simulink library "DAEMOT_Lib"  (R2019b)
settings: Solver=ode45  StartTime=0.0  StopTime=10.0  FixedStep=0.1  RelTol=1e-3
undefined symbols (not defined in the file or in its folder): Controller, CP, Ctrl, Ctrl_Fcn, Elec1, f, F2, Fluid, lag1, Mission, Moody, PropellerProp, rev_comms_sink
libraries: $bdroot x200, instrumentlib x21, simulink x5, dspsigops x2
(part 7 of 13)

== system DAEMOT_Lib/Electrical/Air Vehicle ==
  In1 : Inport
  Bus Creator2 : BusCreator  Inputs=4
  Bus Selector2 : BusSelector  OutputSignals=aspeed,torque
  Constant : Constant  Value=theta
  Data_Sink : Subsystem  LoadFcn=|  InitFcn=|  mask(Data Sink){}
      LoadFcn=|
      | h      = get_param(gcb,'handle');   % Get block handle                           
      | hblock = get(h);     % Parse out handles structure
      | 
      | str = [hblock.Path(numel(bdroot)+2:end), hblock.Name];
      | str(~ismember(str,['A':'Z' 'a':'z' '0':'9' '_'])) = '';                     
      | set_param([gcb, '/global_data_goto'],'GotoTag',['gdata_',str]);
      |                                
      |                                                                                  
      | clear h hblock str
      InitFcn=|
      | h      = get_param(gcb,'handle');   % Get block handle                           
      | hblock = get(h);     % Parse out handles structure
      | 
      | str = [hblock.Path(numel(bdroot)+2:end), hblock.Name];
      | str(~ismember(str,['A':'Z' 'a':'z' '0':'9' '_'])) = '';                     
      | set_param([gcb, '/global_data_goto'],'GotoTag',['gdata_',str]);
      |                                
      |                                                                                  
      | clear h hblock str
      mask help:
      | Input to this block should be a bus signal with named signals.
      |
      | Bus signals sent to this block will be read by the Data Manager.
      | The Data Manager will handle the global routing of signals.
      |
      | This block should be placed under the mask of components.
      settings: CopyFcn=|
      | h      = get_param(gcb,'handle');   % Get block handle
      | hblock = get(h);     % Parse out handles structure
      | 
      | str = [hblock.Path(numel(bdroot)+2:end), hblock.Name];
      | str(~ismember(str,['A':'Z' 'a':'z' '0':'9' '_'])) = '';
      | set_param([gcb, '/global_data_goto'],'GotoTag',['gdata_',str]);
      | 
      | 
      | clear h hblock str
      settings: NameChangeFcn=|
      | h      = get_param(gcb,'handle');   % Get block handle
      | hblock = get(h);     % Parse out handles structure
      | 
      | str = [hblock.Path(numel(bdroot)+2:end), hblock.Name];
      | str(~ismember(str,['A':'Z' 'a':'z' '0':'9' '_'])) = '';
      | set_param([gcb, '/global_data_goto'],'GotoTag',['gdata_',str]);
      | 
      | 
      | clear h hblock str
      mask Display: text(0.25,0.5,'Data Sink')
  Fcn : Fcn  Expr=u(1)*cos(u(2))
  Fcn1 : Fcn  Expr=u(1)*sin(u(2))
  Integrator : Integrator  InitialCondition=v_initial
  Mux : Mux  Inputs=2
  Sink1 : Subsystem  LoadFcn=rev_comms_sink();  InitFcn=rev_comms_sink();  mask(Sink){}
      mask help: Used for sending data to the upstream component.
      settings: CopyFcn=rev_comms_sink();  NameChangeFcn=rev_comms_sink();
      mask Display: text(0.25,0.5,'Sink')
  Terminator1 : Terminator
  speed : MATLAB Function  TreatAsAtomicUnit=on
  wires:
  Constant/1 -> Mux/2
  [v] -> Mux/1
  Mux/1 -> Fcn/1, Fcn1/1
  Fcn1/1 -> Bus Creator2/4  "Vertical Speed [m_s]"
  Fcn/1 -> Bus Creator2/3  "Lateral Speed [m_s]"
  speed/2(tau) -> [tau]
  speed/1(v_dot) -> Integrator/1
  [omega] -> speed/2(omega)
  [tau] -> Bus Creator2/1  "Load Torque [Nm]"
  Bus Creator2/1 -> Data_Sink/1(" ")
  [v] -> Bus Creator2/2  "Vehicle Speed [m_s]"
  Bus Selector2/2 -> Terminator1/1  "<torque>"
  In1/1 -> Bus Selector2/1
  Bus Selector2/1 -> [omega]  "<aspeed>"
  [tau] -> Sink1/1(In1)
  Integrator/1 -> [v]
  [v] -> speed/1(v)

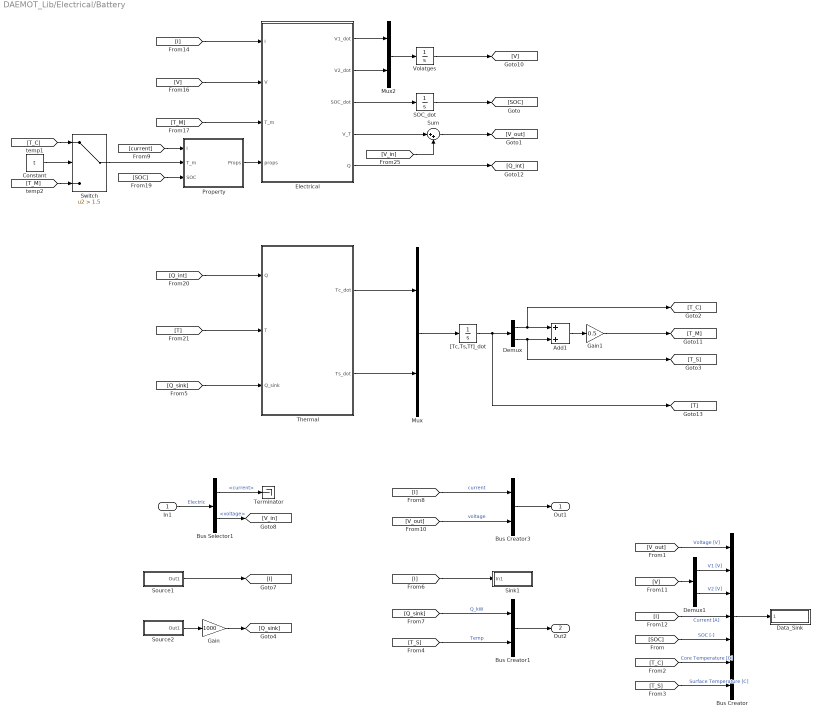
== system DAEMOT_Lib/Electrical/Battery ==
  In1 : Inport
  Add1 : Sum
  Bus Creator : BusCreator  Inputs=7
  Bus Creator1 : BusCreator  Inputs=2
  Bus Creator3 : BusCreator  Inputs=2
  Bus Selector1 : BusSelector  OutputSignals=current,voltage
  Constant : Constant  Value=t
  Data_Sink : Subsystem  LoadFcn=|  InitFcn=|  mask(Data Sink){}
      LoadFcn=|
      | h      = get_param(gcb,'handle');   % Get block handle                           
      | hblock = get(h);     % Parse out handles structure
      | 
      | str = [hblock.Path(numel(bdroot)+2:end), hblock.Name];
      | str(~ismember(str,['A':'Z' 'a':'z' '0':'9' '_'])) = '';                     
      | set_param([gcb, '/global_data_goto'],'GotoTag',['gdata_',str]);
      |                                
      |                                                                                  
      | clear h hblock str
      InitFcn=|
      | h      = get_param(gcb,'handle');   % Get block handle                           
      | hblock = get(h);     % Parse out handles structure
      | 
      | str = [hblock.Path(numel(bdroot)+2:end), hblock.Name];
      | str(~ismember(str,['A':'Z' 'a':'z' '0':'9' '_'])) = '';                     
      | set_param([gcb, '/global_data_goto'],'GotoTag',['gdata_',str]);
      |                                
      |                                                                                  
      | clear h hblock str
      mask help:
      | Input to this block should be a bus signal with named signals.
      |
      | Bus signals sent to this block will be read by the Data Manager.
      | The Data Manager will handle the global routing of signals.
      |
      | This block should be placed under the mask of components.
      settings: CopyFcn=|
      | h      = get_param(gcb,'handle');   % Get block handle
      | hblock = get(h);     % Parse out handles structure
      | 
      | str = [hblock.Path(numel(bdroot)+2:end), hblock.Name];
      | str(~ismember(str,['A':'Z' 'a':'z' '0':'9' '_'])) = '';
      | set_param([gcb, '/global_data_goto'],'GotoTag',['gdata_',str]);
      | 
      | 
      | clear h hblock str
      settings: NameChangeFcn=|
      | h      = get_param(gcb,'handle');   % Get block handle
      | hblock = get(h);     % Parse out handles structure
      | 
      | str = [hblock.Path(numel(bdroot)+2:end), hblock.Name];
      | str(~ismember(str,['A':'Z' 'a':'z' '0':'9' '_'])) = '';
      | set_param([gcb, '/global_data_goto'],'GotoTag',['gdata_',str]);
      | 
      | 
      | clear h hblock str
      mask Display: text(0.25,0.5,'Data Sink')
  Demux : Demux  Outputs=2
  Demux1 : Demux  Outputs=2
  Electrical : MATLAB Function  TreatAsAtomicUnit=on
  Gain : Gain  Gain=1000
  Gain1 : Gain  Gain=0.5
  Mux : Mux  Inputs=2
  Mux2 : Mux  Inputs=2
  Property : Subsystem
  SOC_dot : Integrator  InitialCondition=SOC_initial
  Sink1 : Subsystem  LoadFcn=rev_comms_sink();  InitFcn=rev_comms_sink();  mask(Sink){}
      mask help: Used for sending data to the upstream component.
      settings: CopyFcn=rev_comms_sink();  NameChangeFcn=rev_comms_sink();
      mask Display: text(0.25,0.5,'Sink')
  Source1 : Subsystem  mask(Source){}
      mask help: Used for receiving data from the downstream component.
      mask init:
      | n_src = gcb;
      | n_src = str2num(n_src(end));
      | try
      |     rev_comms_source(n_src);
      | catch
      | 
      | end
      mask Display: text(0.25,0.5,'Source')
  Source2 : Subsystem  mask(Source){}
      mask help: Used for receiving data from the downstream component.
      mask init:
      | n_src = gcb;
      | n_src = str2num(n_src(end));
      | try
      |     rev_comms_source(n_src);
      | catch
      | 
      | end
      mask Display: text(0.25,0.5,'Source')
  Sum : Sum  Inputs=|++
  Switch : Switch  Criteria=u2 > Threshold  Threshold=1.5
  Terminator : Terminator
  Thermal : MATLAB Function  TreatAsAtomicUnit=on
  Volatges : Integrator  InitialCondition=RC_initial
  "[Tc,Ts,Tf]_dot" : Integrator  InitialCondition=[Tc_initial, Ts_initial]
  Out1 : Outport
  Out2 : Outport  Port=2
  wires:
  [I] -> Bus Creator/4  "Current [A]"
  [V] -> Demux1/1
  Demux1/1 -> Bus Creator/2  "V1 [V]"
  Demux1/2 -> Bus Creator/3  "V2 [V]"
  Switch/1 -> Property/2(T_m)
  [T_M] -> Switch/3
  [T_C] -> Switch/1
  Constant/1 -> Switch/2
  Electrical/2(V2_dot) -> Mux2/2
  Electrical/1(V1_dot) -> Mux2/1
  Electrical/3(SOC_dot) -> SOC_dot/1
  Sum/1 -> [V_out]
  Electrical/4(V_T) -> Sum/1
  [V_in] -> Sum/2
  Electrical/5(Q) -> [Q_int]
  Property/1(Props) -> Electrical/4(props)
  [V] -> Electrical/2(V)
  [T_M] -> Electrical/3(T_m)
  [I] -> Electrical/1(I)
  Mux2/1 -> Volatges/1
  Demux/2 -> [T_S], Add1/2
  Demux/1 -> [T_C], Add1/1
  "[Tc,Ts,Tf]_dot"/1 -> [T], Demux/1
  SOC_dot/1 -> [SOC]
  Volatges/1 -> [V]
  Add1/1 -> Gain1/1
  Mux/1 -> "[Tc,Ts,Tf]_dot"/1
  [SOC] -> Bus Creator/5  "SOC [-]"
  [V_out] -> Bus Creator/1  "Voltage [V]"
  [T_C] -> Bus Creator/6  "Core Temperature [C]"
  [T_S] -> Bus Creator/7  "Surface Temperature [C]"
  In1/1 -> Bus Selector1/1  "Electric"
  Bus Creator3/1 -> Out1/1
  [I] -> Bus Creator3/1  "current"
  Bus Selector1/1 -> Terminator/1  "<current>"
  Bus Selector1/2 -> [V_in]  "<voltage>"
  [V_out] -> Bus Creator3/2  "voltage"
  [current] -> Property/1(I)
  Gain1/1 -> [T_M]
  Bus Creator/1 -> Data_Sink/1(" ")
  [SOC] -> Property/3(SOC)
  [Q_int] -> Thermal/1(Q)
  [T] -> Thermal/2(T)
  Thermal/1(Tc_dot) -> Mux/1
  Thermal/2(Ts_dot) -> Mux/2
  [Q_sink] -> Thermal/3(Q_sink)
  Source2/1(Out1) -> Gain/1
  [I] -> Sink1/1(In1)
  Source1/1(Out1) -> [I]
  Bus Creator1/1 -> Out2/1
  [T_S] -> Bus Creator1/2  "Temp"
  [Q_sink] -> Bus Creator1/1  "Q_kW"
  Gain/1 -> [Q_sink]

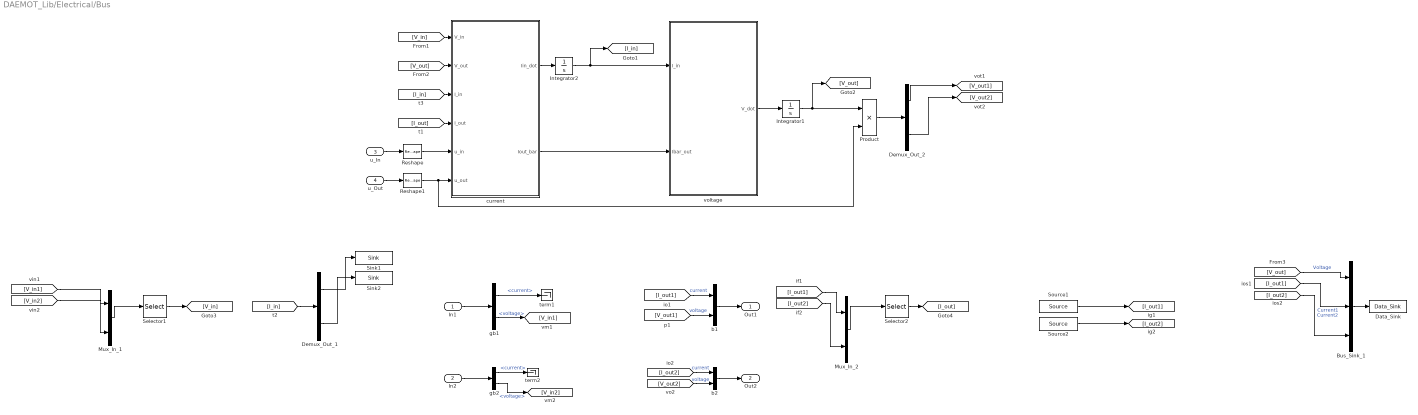
== system DAEMOT_Lib/Electrical/Bus ==
  In1 : Inport
  In2 : Inport  Port=2
  u_In : Inport  Port=3
  u_Out : Inport  Port=4
  Bus_Sink_1 : BusCreator  Inputs=3
  Data_Sink : $bdroot/Support Functions/Data_Sink
  Demux_Out_1 : Demux  Outputs=2
  Demux_Out_2 : Demux  Outputs=2
  Integrator1 : Integrator  InitialCondition=V_initial
  Integrator2 : Integrator  InitialCondition=I_initial*ones(Num_In,1)
  Mux_In_1 : Mux  Inputs=2
  Mux_In_2 : Mux  Inputs=2
  Product : Product
  Reshape : Reshape
  Reshape1 : Reshape
  Selector1 : Selector  InputPortWidth=2  IndexOptions=Index vector (dialog)  Indices=[1 2 ]  OutputSizes=1
  Selector2 : Selector  InputPortWidth=2  IndexOptions=Index vector (dialog)  Indices=[1 2 ]  OutputSizes=1
  Sink1 : $bdroot/Support Functions/Sink
  Sink2 : $bdroot/Support Functions/Sink
  Source1 : $bdroot/Support Functions/Source
  Source2 : $bdroot/Support Functions/Source
  b1 : BusCreator  Inputs=2
  b2 : BusCreator  Inputs=2
  current : MATLAB Function  TreatAsAtomicUnit=on
  gb1 : BusSelector  OutputSignals=current,voltage
  gb2 : BusSelector  OutputSignals=current,voltage
  term1 : Terminator
  term2 : Terminator
  voltage : MATLAB Function  TreatAsAtomicUnit=on
  Out1 : Outport  VectorParamsAs1DForOutWhenUnconnected=off
  Out2 : Outport  Port=2  VectorParamsAs1DForOutWhenUnconnected=off
  wires:
  Demux_Out_1/1 -> Sink1/1
  [V_in1] -> Mux_In_1/1
  gb1/2 -> [V_in1]  "<voltage>"
  gb1/1 -> term1/1  "<current>"
  In1/1 -> gb1/1
  [I_in] -> Demux_Out_1/1
  Integrator2/1 -> voltage/1(I_in), [I_in]
  voltage/1(V_dot) -> Integrator1/1
  Integrator1/1 -> Product/1, [V_out]
  [V_out] -> current/2(V_out)
  Mux_In_1/1 -> Selector1/1
  current/1(Iin_dot) -> Integrator2/1
  [I_in] -> current/3(I_in)
  u_In/1 -> Reshape/1
  Demux_Out_2/1 -> [V_out1]
  Bus_Sink_1/1 -> Data_Sink/1
  [I_out1] -> Mux_In_2/1
  Mux_In_2/1 -> Selector2/1
  [V_out1] -> b1/2  "voltage"
  [I_out1] -> b1/1  "current"
  Source1/1 -> [I_out1]
  b1/1 -> Out1/1
  u_Out/1 -> Reshape1/1
  current/2(Iout_bar) -> voltage/2(Ibar_out)
  Product/1 -> Demux_Out_2/1
  [V_in] -> current/1(V_in)
  Selector1/1 -> [V_in]
  In2/1 -> gb2/1
  gb2/2 -> [V_in2]  "<voltage>"
  gb2/1 -> term2/1  "<current>"
  Demux_Out_1/2 -> Sink2/1
  [V_in2] -> Mux_In_1/2
  [I_out] -> current/4(I_out)
  Selector2/1 -> [I_out]
  [V_out] -> Bus_Sink_1/1  "Voltage"
  [I_out1] -> Bus_Sink_1/2  "Current1"
  [I_out2] -> b2/1  "current"
  [V_out2] -> b2/2  "voltage"
  [I_out2] -> Bus_Sink_1/3  "Current2"
  b2/1 -> Out2/1
  Source2/1 -> [I_out2]
  [I_out2] -> Mux_In_2/2
  Demux_Out_2/2 -> [V_out2]
  Reshape/1 -> current/5(u_in)
  Reshape1/1 -> Product/2, current/6(u_out)

== system DAEMOT_Lib/Electrical/Capacitor ==
  In1 : Inport
  Bus Creator1 : BusCreator  Inputs=1
  Bus Creator3 : BusCreator  Inputs=2
  Bus Selector1 : BusSelector  OutputSignals=current,voltage
  Data_Sink : $bdroot/Support Functions/Data_Sink
  Integrator2 : Integrator  InitialCondition=V_initial
  Sink1 : $bdroot/Support Functions/Sink
  Source1 : $bdroot/Support Functions/Source
  Terminator : Terminator
  Voltage : MATLAB Function  TreatAsAtomicUnit=on
  Out1 : Outport  VectorParamsAs1DForOutWhenUnconnected=off
  wires:
  Integrator2/1 -> [V]
  [Current_out] -> Bus Creator3/1  "current"
  Bus Selector1/1 -> [Current_in]  "<current>"
  Bus Selector1/2 -> Terminator/1  "<voltage>"
  [V] -> Bus Creator3/2  "voltage"
  [V] -> Sink1/1
  In1/1 -> Bus Selector1/1  "electric"
  [Current_out] -> Voltage/2(I_out)
  Bus Creator3/1 -> Out1/1
  Voltage/1(V_dot) -> Integrator2/1
  [Current_in] -> Voltage/1(I_in)
  [V] -> Bus Creator1/1  "Voltage"
  Bus Creator1/1 -> Data_Sink/1
  Source1/1 -> [Current_out]

== system DAEMOT_Lib/Electrical/Converter ==
  In1 : Inport
  In2 : Inport  Port=2
  In3 : Inport  Port=3
  Bus Creator1 : BusCreator  Inputs=2
  Bus Creator2 : BusCreator  Inputs=3
  Bus Creator3 : BusCreator  Inputs=2
  Bus Selector1 : BusSelector  OutputSignals=current,voltage
  Current : MATLAB Function  TreatAsAtomicUnit=on
  Data_Sink : $bdroot/Support Functions/Data_Sink
  Gain : Gain  Gain=1000
  Integrator1 : Integrator  InitialCondition=T_initial
  Scope : Scope
  Sink1 : $bdroot/Support Functions/Sink
  Source1 : $bdroot/Support Functions/Source
  Source2 : $bdroot/Support Functions/Source
  Terminator : Terminator
  Thermal : MATLAB Function  TreatAsAtomicUnit=on
  Voltage : MATLAB Function  TreatAsAtomicUnit=on
  Out1 : Outport  VectorParamsAs1DForOutWhenUnconnected=off
  Out2 : Outport  Port=2  VectorParamsAs1DForOutWhenUnconnected=off
  wires:
  Source2/1 -> Gain/1
  Voltage/2(Q) -> Scope/1, [Q]
  [I_out] -> Voltage/3(I_out)
  [T] -> Bus Creator2/3  "Temperature"
  [I_out] -> Bus Creator2/1  "Current"
  [V_out] -> Bus Creator2/2  "Voltage"
  Bus Creator2/1 -> Data_Sink/1
  Thermal/1(T_dot) -> Integrator1/1
  Integrator1/1 -> [T]
  [Q] -> Thermal/1(Q)
  [Q_sink] -> Thermal/2(Q_sink)
  In3/1 -> Current/3(s), Voltage/5(s)
  In2/1 -> Current/2(D), Voltage/4(D)
  Current/1(I_in) -> [I_in], Voltage/2(I_in)
  [I_out] -> Current/1(I_out)
  Voltage/1(V_out) -> [V_out]
  [V_in] -> Voltage/1(V_in)
  [I_out] -> Bus Creator3/1  "current"
  Source1/1 -> [I_out]
  Bus Selector1/1 -> Terminator/1  "<current>"
  Bus Selector1/2 -> [V_in]  "<voltage>"
  [V_out] -> Bus Creator3/2  "voltage"
  In1/1 -> Bus Selector1/1  "electric"
  Bus Creator3/1 -> Out1/1
  [I_in] -> Sink1/1
  Bus Creator1/1 -> Out2/1
  [T] -> Bus Creator1/2  "Temp"
  [Q_sink] -> Bus Creator1/1  "Q_kW"
  Gain/1 -> [Q_sink]

== system DAEMOT_Lib/Electrical/Cooling Sink ==
  In1 : Inport
  In2 : Inport  Port=2
  Sink1 : $bdroot/Support Functions/Sink
  Terminator : Terminator
  wires:
  In1/1 -> Terminator/1
  In2/1 -> Sink1/1  "Q_kW"

== system DAEMOT_Lib/Electrical/Cooling Source ==
  In1 : Inport
  Constant : Constant
  Source1 : $bdroot/Support Functions/Source
  Terminator : Terminator
  b1 : BusCreator  Inputs=2
  Out1 : Outport  VectorParamsAs1DForOutWhenUnconnected=off
  wires:
  In1/1 -> b1/1  "Q_kW"
  b1/1 -> Out1/1
  Constant/1 -> b1/2  "Temp"
  Source1/1 -> Terminator/1

== system DAEMOT_Lib/Electrical/Current Sink ==
  In1 : Inport
  In2 : Inport  Port=2
  Sink1 : Subsystem  LoadFcn=rev_comms_sink();  InitFcn=rev_comms_sink();  mask(Sink){}
      mask help: Used for sending data to the upstream component.
      settings: CopyFcn=rev_comms_sink();  NameChangeFcn=rev_comms_sink();
      mask Display: text(0.25,0.5,'Sink')
  Terminator : Terminator
  wires:
  In1/1 -> Terminator/1
  In2/1 -> Sink1/1(In1)  "current"

== system DAEMOT_Lib/Electrical/Current Source ==
  In1 : Inport
  Constant : Constant  Value=0
  Source1 : Subsystem  mask(Source){}
      mask help: Used for receiving data from the downstream component.
      mask init:
      | n_src = gcb;
      | n_src = str2num(n_src(end));
      | try
      |     rev_comms_source(n_src);
      | catch
      | 
      | end
      mask Display: text(0.25,0.5,'Source')
  Terminator : Terminator
  b1 : BusCreator  Inputs=2
  Out1 : Outport  VectorParamsAs1DForOutWhenUnconnected=off
  wires:
  b1/1 -> Out1/1
  Constant/1 -> b1/2  "voltage"
  Source1/1(Out1) -> Terminator/1
  In1/1 -> b1/1  "current"

== system DAEMOT_Lib/Electrical/ESC ==
  In1 : Inport
  Bus Creator2 : BusCreator  Inputs=1
  Bus Selector2 : BusSelector  OutputSignals=current,voltage
  Data_Sink : Subsystem  LoadFcn=|  InitFcn=|  mask(Data Sink){}
      LoadFcn=|
      | h      = get_param(gcb,'handle');   % Get block handle                           
      | hblock = get(h);     % Parse out handles structure
      | 
      | str = [hblock.Path(numel(bdroot)+2:end), hblock.Name];
      | str(~ismember(str,['A':'Z' 'a':'z' '0':'9' '_'])) = '';                     
      | set_param([gcb, '/global_data_goto'],'GotoTag',['gdata_',str]);
      |                                
      |                                                                                  
      | clear h hblock str
      InitFcn=|
      | h      = get_param(gcb,'handle');   % Get block handle                           
      | hblock = get(h);     % Parse out handles structure
      | 
      | str = [hblock.Path(numel(bdroot)+2:end), hblock.Name];
      | str(~ismember(str,['A':'Z' 'a':'z' '0':'9' '_'])) = '';                     
      | set_param([gcb, '/global_data_goto'],'GotoTag',['gdata_',str]);
      |                                
      |                                                                                  
      | clear h hblock str
      mask help:
      | Input to this block should be a bus signal with named signals.
      |
      | Bus signals sent to this block will be read by the Data Manager.
      | The Data Manager will handle the global routing of signals.
      |
      | This block should be placed under the mask of components.
      settings: CopyFcn=|
      | h      = get_param(gcb,'handle');   % Get block handle
      | hblock = get(h);     % Parse out handles structure
      | 
      | str = [hblock.Path(numel(bdroot)+2:end), hblock.Name];
      | str(~ismember(str,['A':'Z' 'a':'z' '0':'9' '_'])) = '';
      | set_param([gcb, '/global_data_goto'],'GotoTag',['gdata_',str]);
      | 
      | 
      | clear h hblock str
      settings: NameChangeFcn=|
      | h      = get_param(gcb,'handle');   % Get block handle
      | hblock = get(h);     % Parse out handles structure
      | 
      | str = [hblock.Path(numel(bdroot)+2:end), hblock.Name];
      | str(~ismember(str,['A':'Z' 'a':'z' '0':'9' '_'])) = '';
      | set_param([gcb, '/global_data_goto'],'GotoTag',['gdata_',str]);
      | 
      | 
      | clear h hblock str
      mask Display: text(0.25,0.5,'Data Sink')
  Polynomial : Polyval  Coefs=Esc.coeffs
  Sink1 : Subsystem  LoadFcn=rev_comms_sink();  InitFcn=rev_comms_sink();  mask(Sink){}
      mask help: Used for sending data to the upstream component.
      settings: CopyFcn=rev_comms_sink();  NameChangeFcn=rev_comms_sink();
      mask Display: text(0.25,0.5,'Sink')
  Terminator1 : Terminator
  wires:
  [current] -> Sink1/1(In1)
  Bus Selector2/2 -> [voltage]  "<voltage>"
  In1/1 -> Bus Selector2/1
  Bus Creator2/1 -> Data_Sink/1(" ")
  [current] -> Bus Creator2/1  "Current Load [A]"
  Bus Selector2/1 -> Terminator1/1  "<current>"
  [voltage] -> Polynomial/1
  Polynomial/1 -> [current]

== system DAEMOT_Lib/Electrical/Effort Sink ==
  In1 : Inport
  Sink1 : Subsystem  LoadFcn=rev_comms_sink();  InitFcn=rev_comms_sink();  mask(Sink){}
      mask help: Used for sending data to the upstream component.
      settings: CopyFcn=rev_comms_sink();  NameChangeFcn=rev_comms_sink();
      mask Display: text(0.25,0.5,'Sink')
  Terminator : Terminator
  val : Constant  Value=value
  wires:
  val/1 -> Sink1/1(In1)
  In1/1 -> Terminator/1

== system DAEMOT_Lib/Electrical/Effort Source ==
  Constant : Constant  Value=0
  Source1 : Subsystem  mask(Source){}
      mask help: Used for receiving data from the downstream component.
      mask init:
      | n_src = gcb;
      | n_src = str2num(n_src(end));
      | try
      |     rev_comms_source(n_src);
      | catch
      | 
      | end
      mask Display: text(0.25,0.5,'Source')
  Terminator : Terminator
  b1 : BusCreator  Inputs=2
  val : Constant  Value=value
  Out1 : Outport  VectorParamsAs1DForOutWhenUnconnected=off
  wires:
  val/1 -> b1/2  "voltage"
  Constant/1 -> b1/1  "current"
  Source1/1(Out1) -> Terminator/1
  b1/1 -> Out1/1

== system DAEMOT_Lib/Electrical/Engine ==
  In1 : Inport
  In2 : Inport  Port=2
  Bus Creator1 : BusCreator  Inputs=2
  Bus Selector1 : BusSelector  OutputSignals=current,voltage
  Compare To Constant : simulink/Logic and Bit Operations/Compare To Constant  relop=>  const=.01  OutDataTypeStr=uint8
  Constant : Constant  Value=0
  Data_Sink : Subsystem  LoadFcn=|  InitFcn=|  mask(Data Sink){}
      LoadFcn=|
      | h      = get_param(gcb,'handle');   % Get block handle                           
      | hblock = get(h);     % Parse out handles structure
      | 
      | str = [hblock.Path(numel(bdroot)+2:end), hblock.Name];
      | str(~ismember(str,['A':'Z' 'a':'z' '0':'9' '_'])) = '';                     
      | set_param([gcb, '/global_data_goto'],'GotoTag',['gdata_',str]);
      |                                
      |                                                                                  
      | clear h hblock str
      InitFcn=|
      | h      = get_param(gcb,'handle');   % Get block handle                           
      | hblock = get(h);     % Parse out handles structure
      | 
      | str = [hblock.Path(numel(bdroot)+2:end), hblock.Name];
      | str(~ismember(str,['A':'Z' 'a':'z' '0':'9' '_'])) = '';                     
      | set_param([gcb, '/global_data_goto'],'GotoTag',['gdata_',str]);
      |                                
      |                                                                                  
      | clear h hblock str
      mask help:
      | Input to this block should be a bus signal with named signals.
      |
      | Bus signals sent to this block will be read by the Data Manager.
      | The Data Manager will handle the global routing of signals.
      |
      | This block should be placed under the mask of components.
      settings: CopyFcn=|
      | h      = get_param(gcb,'handle');   % Get block handle
      | hblock = get(h);     % Parse out handles structure
      | 
      | str = [hblock.Path(numel(bdroot)+2:end), hblock.Name];
      | str(~ismember(str,['A':'Z' 'a':'z' '0':'9' '_'])) = '';
      | set_param([gcb, '/global_data_goto'],'GotoTag',['gdata_',str]);
      | 
      | 
      | clear h hblock str
      settings: NameChangeFcn=|
      | h      = get_param(gcb,'handle');   % Get block handle
      | hblock = get(h);     % Parse out handles structure
      | 
      | str = [hblock.Path(numel(bdroot)+2:end), hblock.Name];
      | str(~ismember(str,['A':'Z' 'a':'z' '0':'9' '_'])) = '';
      | set_param([gcb, '/global_data_goto'],'GotoTag',['gdata_',str]);
      | 
      | 
      | clear h hblock str
      mask Display: text(0.25,0.5,'Data Sink')
  Dynamic Saturation : Subsystem
  Fcn1 : Fcn  Expr="S_coeffs(1)*u(2)^2 + S_coeffs(2)*u(1)^2 + S_coeffs(3) +  S_coeffs(4)*u(1)*u(2) + S_coeffs(5)*u(2) +  S_coeffs(6)*u(1);"
  Gain : Gain  Gain=G
  Gain1 : Gain  Gain=1/G
  Gain2 : Gain  Gain=1/tau
  Gain3 : Gain  Gain=I_coeffs(2)
  Gain4 : Gain  Gain=-1
  Integrator : Integrator
  Mux1 : Mux  Inputs=2
  Mux3 : Mux  Inputs=2
  Polynomial1 : Polyval  Coefs=B_coeffs
  Product : Product
  Scope : Scope
  Scope2 : Scope
  Sink1 : Subsystem  LoadFcn=rev_comms_sink();  InitFcn=rev_comms_sink();  mask(Sink){}
      mask help: Used for sending data to the upstream component.
      settings: CopyFcn=rev_comms_sink();  NameChangeFcn=rev_comms_sink();
      mask Display: text(0.25,0.5,'Sink')
  Sum : Sum  Inputs=|+-
  Terminator1 : Terminator
  wires:
  Gain/1 -> Sum/1, Scope/1
  [voltage] -> Mux1/1
  Gain1/1 -> Mux1/2
  Mux1/1 -> Fcn1/1
  Gain3/1 -> Gain/1
  Integrator/1 -> [current]
  [voltage] -> Polynomial1/1
  Polynomial1/1 -> Dynamic Saturation/1(up)
  Constant/1 -> Dynamic Saturation/3(dn)
  [u] -> Mux3/1, Dynamic Saturation/2(u)
  Gain2/1 -> Integrator/1
  Sum/1 -> Gain2/1
  [current] -> Sum/2
  Bus Selector1/2 -> [voltage]  "<voltage>"
  Bus Selector1/1 -> Terminator1/1  "<current>"
  [current] -> Sink1/1(In1)
  In1/1 -> Bus Selector1/1  "Electrical"
  [current] -> Bus Creator1/1  "Current [A]"
  Bus Creator1/1 -> Data_Sink/1(" ")
  In2/1 -> [u]
  [SFC] -> Bus Creator1/2  "SFC [g_kW-h]"
  Dynamic Saturation/1(Out1) -> Mux3/2, Gain3/1
  [current] -> Gain4/1, Gain1/1
  Gain4/1 -> Compare To Constant/1
  Compare To Constant/1 -> Product/2
  Product/1 -> [SFC]
  Fcn1/1 -> Product/1
  Mux3/1 -> Scope2/1

== system DAEMOT_Lib/Electrical/Gearbox ==
  In1 : Inport
  Bus Creator2 : BusCreator  Inputs=2
  Bus Creator3 : BusCreator  Inputs=2
  Bus Selector1 : BusSelector  OutputSignals=aspeed,torque
  Data_Sink : Subsystem  LoadFcn=|  InitFcn=|  mask(Data Sink){}
      LoadFcn=|
      | h      = get_param(gcb,'handle');   % Get block handle                           
      | hblock = get(h);     % Parse out handles structure
      | 
      | str = [hblock.Path(numel(bdroot)+2:end), hblock.Name];
      | str(~ismember(str,['A':'Z' 'a':'z' '0':'9' '_'])) = '';                     
      | set_param([gcb, '/global_data_goto'],'GotoTag',['gdata_',str]);
      |                                
      |                                                                                  
      | clear h hblock str
      InitFcn=|
      | h      = get_param(gcb,'handle');   % Get block handle                           
      | hblock = get(h);     % Parse out handles structure
      | 
      | str = [hblock.Path(numel(bdroot)+2:end), hblock.Name];
      | str(~ismember(str,['A':'Z' 'a':'z' '0':'9' '_'])) = '';                     
      | set_param([gcb, '/global_data_goto'],'GotoTag',['gdata_',str]);
      |                                
      |                                                                                  
      | clear h hblock str
      mask help:
      | Input to this block should be a bus signal with named signals.
      |
      | Bus signals sent to this block will be read by the Data Manager.
      | The Data Manager will handle the global routing of signals.
      |
      | This block should be placed under the mask of components.
      settings: CopyFcn=|
      | h      = get_param(gcb,'handle');   % Get block handle
      | hblock = get(h);     % Parse out handles structure
      | 
      | str = [hblock.Path(numel(bdroot)+2:end), hblock.Name];
      | str(~ismember(str,['A':'Z' 'a':'z' '0':'9' '_'])) = '';
      | set_param([gcb, '/global_data_goto'],'GotoTag',['gdata_',str]);
      | 
      | 
      | clear h hblock str
      settings: NameChangeFcn=|
      | h      = get_param(gcb,'handle');   % Get block handle
      | hblock = get(h);     % Parse out handles structure
      | 
      | str = [hblock.Path(numel(bdroot)+2:end), hblock.Name];
      | str(~ismember(str,['A':'Z' 'a':'z' '0':'9' '_'])) = '';
      | set_param([gcb, '/global_data_goto'],'GotoTag',['gdata_',str]);
      | 
      | 
      | clear h hblock str
      mask Display: text(0.25,0.5,'Data Sink')
  Sink1 : Subsystem  LoadFcn=rev_comms_sink();  InitFcn=rev_comms_sink();  mask(Sink){}
      mask help: Used for sending data to the upstream component.
      settings: CopyFcn=rev_comms_sink();  NameChangeFcn=rev_comms_sink();
      mask Display: text(0.25,0.5,'Sink')
  Source1 : Subsystem  mask(Source){}
      mask help: Used for receiving data from the downstream component.
      mask init:
      | n_src = gcb;
      | n_src = str2num(n_src(end));
      | try
      |     rev_comms_source(n_src);
      | catch
      | 
      | end
      mask Display: text(0.25,0.5,'Source')
  downstream : MATLAB Function  TreatAsAtomicUnit=on
  upstream : MATLAB Function  TreatAsAtomicUnit=on
  Out1 : Outport
  wires:
  [var_in] -> downstream/1(var_in)
  downstream/1(var_out) -> [var_out]
  Bus Creator2/1 -> Data_Sink/1(" ")
  upstream/1(out_up) -> [out_up]
  [in_down] -> upstream/1(in_down)
  [out_up] -> Sink1/1(In1)
  Bus Creator3/1 -> Out1/1
  In1/1 -> Bus Selector1/1  "mechacnical"
  [var_out] -> Bus Creator3/2  "torque"
  Bus Selector1/2 -> [var_in]  "<torque>"
  Bus Selector1/1 -> [term]  "<aspeed>"
  Source1/1(Out1) -> [in_down]
  [in_down] -> Bus Creator3/1  "aspeed"
  [var_out] -> Bus Creator2/2  "Output Torque [Nm]"
  [out_up] -> Bus Creator2/1  "Input Speed [rad_s]"

== system DAEMOT_Lib/Electrical/Generator ==
  In1 : Inport
  In2 : Inport  Port=2
  Bus Creator1 : BusCreator  Inputs=2
  Bus Selector1 : BusSelector  OutputSignals=current,voltage
  Data_Sink : $bdroot/Support Functions/Data_Sink
  Sink1 : $bdroot/Support Functions/Sink
  Terminator : Terminator
  Voltage1 : MATLAB Function  TreatAsAtomicUnit=on
  wires:
  [SFC] -> Bus Creator1/2  "SFC"
  Voltage1/2(S) -> [SFC]
  In2/1 -> [u]
  Bus Creator1/1 -> Data_Sink/1
  [I] -> Bus Creator1/1  "Current"
  In1/1 -> Bus Selector1/1  "electric"
  [I] -> Sink1/1
  Bus Selector1/2 -> [V]  "<voltage>"
  Bus Selector1/1 -> Terminator/1  "<current>"
  [V] -> Voltage1/1(V_in)
  [u] -> Voltage1/2(u)
  Voltage1/1(I) -> [I]

== system DAEMOT_Lib/Electrical/Ground Vehicle ==
  In1 : Inport
  In2 : Inport  Port=2
  Bus Creator1 : BusCreator  Inputs=2
  Bus Selector1 : BusSelector  OutputSignals=torque,speed
  Data_Sink : $bdroot/Support Functions/Data_Sink
  Sink1 : $bdroot/Support Functions/Sink
  Terminator : Terminator
  Torque : MATLAB Function  TreatAsAtomicUnit=on
  wires:
  Torque/2(v) -> [v]
  Bus Creator1/1 -> Data_Sink/1
  [t_brake] -> Torque/2(t_brake)
  In2/1 -> [t_brake]
  [v] -> Bus Creator1/2  "Vehicle Speed"
  In1/1 -> Bus Selector1/1  "mechanical"
  Bus Selector1/2 -> [omega]  "<speed>"
  Bus Selector1/1 -> Terminator/1  "<torque>"
  [omega] -> Torque/1(omega)
  Torque/1(t_load) -> [tau_load]
  [tau_load] -> Sink1/1, Bus Creator1/1  "Load Torque"

== system DAEMOT_Lib/Electrical/Inductor ==
  In1 : Inport
  Bus Creator1 : BusCreator  Inputs=1
  Bus Creator3 : BusCreator  Inputs=2
  Bus Selector1 : BusSelector  OutputSignals=current,voltage
  Current : MATLAB Function  TreatAsAtomicUnit=on
  Data_Sink : $bdroot/Support Functions/Data_Sink
  Integrator3 : Integrator  InitialCondition=I_initial
  Sink1 : $bdroot/Support Functions/Sink
  Source1 : $bdroot/Support Functions/Source
  Terminator : Terminator
  Out1 : Outport  VectorParamsAs1DForOutWhenUnconnected=off
  wires:
  Bus Creator3/1 -> Out1/1
  In1/1 -> Bus Selector1/1  "electric"
  [I] -> Sink1/1
  [V_out] -> Bus Creator3/2  "voltage"
  Bus Selector1/2 -> [V_in]  "<voltage>"
  Bus Selector1/1 -> Terminator/1  "<current>"
  Source1/1 -> [V_out]
  [I] -> Bus Creator3/1  "current"
  [V_in] -> Current/1(V_in)
  [V_out] -> Current/2(V_out)
  Current/1(dI_dt) -> Integrator3/1
  Integrator3/1 -> [I]
  Bus Creator1/1 -> Data_Sink/1
  [I] -> Bus Creator1/1  "Current"

== system DAEMOT_Lib/Electrical/Inverter ==
  In1 : Inport
  In2 : Inport  Port=2
  Bus Creator1 : BusCreator  Inputs=2
  Bus Creator2 : BusCreator  Inputs=3
  Bus Creator3 : BusCreator  Inputs=2
  Bus Selector1 : BusSelector  OutputSignals=current,voltage
  Current : MATLAB Function  TreatAsAtomicUnit=on
  Data_Sink : Subsystem  LoadFcn=|  InitFcn=|  mask(Data Sink){}
      LoadFcn=|
      | h      = get_param(gcb,'handle');   % Get block handle                           
      | hblock = get(h);     % Parse out handles structure
      | 
      | str = [hblock.Path(numel(bdroot)+2:end), hblock.Name];
      | str(~ismember(str,['A':'Z' 'a':'z' '0':'9' '_'])) = '';                     
      | set_param([gcb, '/global_data_goto'],'GotoTag',['gdata_',str]);
      |                                
      |                                                                                  
      | clear h hblock str
      InitFcn=|
      | h      = get_param(gcb,'handle');   % Get block handle                           
      | hblock = get(h);     % Parse out handles structure
      | 
      | str = [hblock.Path(numel(bdroot)+2:end), hblock.Name];
      | str(~ismember(str,['A':'Z' 'a':'z' '0':'9' '_'])) = '';                     
      | set_param([gcb, '/global_data_goto'],'GotoTag',['gdata_',str]);
      |                                
      |                                                                                  
      | clear h hblock str
      mask help:
      | Input to this block should be a bus signal with named signals.
      |
      | Bus signals sent to this block will be read by the Data Manager.
      | The Data Manager will handle the global routing of signals.
      |
      | This block should be placed under the mask of components.
      settings: CopyFcn=|
      | h      = get_param(gcb,'handle');   % Get block handle
      | hblock = get(h);     % Parse out handles structure
      | 
      | str = [hblock.Path(numel(bdroot)+2:end), hblock.Name];
      | str(~ismember(str,['A':'Z' 'a':'z' '0':'9' '_'])) = '';
      | set_param([gcb, '/global_data_goto'],'GotoTag',['gdata_',str]);
      | 
      | 
      | clear h hblock str
      settings: NameChangeFcn=|
      | h      = get_param(gcb,'handle');   % Get block handle
      | hblock = get(h);     % Parse out handles structure
      | 
      | str = [hblock.Path(numel(bdroot)+2:end), hblock.Name];
      | str(~ismember(str,['A':'Z' 'a':'z' '0':'9' '_'])) = '';
      | set_param([gcb, '/global_data_goto'],'GotoTag',['gdata_',str]);
      | 
      | 
      | clear h hblock str
      mask Display: text(0.25,0.5,'Data Sink')
  Gain : Gain  Gain=1000
  Integrator1 : Integrator  InitialCondition=T_initial
  Scope : Scope
  Sink1 : Subsystem  LoadFcn=rev_comms_sink();  InitFcn=rev_comms_sink();  mask(Sink){}
      mask help: Used for sending data to the upstream component.
      settings: CopyFcn=rev_comms_sink();  NameChangeFcn=rev_comms_sink();
      mask Display: text(0.25,0.5,'Sink')
  Source1 : Subsystem  mask(Source){}
      mask help: Used for receiving data from the downstream component.
      mask init:
      | n_src = gcb;
      | n_src = str2num(n_src(end));
      | try
      |     rev_comms_source(n_src);
      | catch
      | 
      | end
      mask Display: text(0.25,0.5,'Source')
  Source2 : Subsystem  mask(Source){}
      mask help: Used for receiving data from the downstream component.
      mask init:
      | n_src = gcb;
      | n_src = str2num(n_src(end));
      | try
      |     rev_comms_source(n_src);
      | catch
      | 
      | end
      mask Display: text(0.25,0.5,'Source')
  Terminator : Terminator
  Thermal : MATLAB Function  TreatAsAtomicUnit=on
  Voltage : MATLAB Function  TreatAsAtomicUnit=on
  Out1 : Outport
  Out2 : Outport  Port=2
  tag scope: Q_inv=global
  wires:
  [V_in] -> Voltage/1(V_in)
  Voltage/1(V_out) -> [V_out]
  [I_out] -> Current/1(I_out)
  Current/1(I_in) -> [I_in]
  In2/1 -> Voltage/3(D), Current/2(D)
  [I_out] -> Voltage/2(I_out)
  Voltage/2(Q) -> [Q], Scope/1
  Bus Creator3/1 -> Out1/1
  In1/1 -> Bus Selector1/1  "electric"
  [I_in] -> Sink1/1(In1)
  [V_out] -> Bus Creator3/2  "voltage"
  Bus Selector1/2 -> [V_in]  "<voltage>"
  Bus Selector1/1 -> Terminator/1  "<current>"
  Source1/1(Out1) -> [I_out]
  [I_out] -> Bus Creator3/1  "current"
  [Q_sink] -> Thermal/2(Q_sink)
  [Q] -> [Q_inv], Thermal/1(Q)
  Integrator1/1 -> [T]
  Thermal/1(T_dot) -> Integrator1/1
  Bus Creator2/1 -> Data_Sink/1(" ")
  [V_out] -> Bus Creator2/2  "Voltage Out [V]"
  [I_in] -> Bus Creator2/1  "Current In [A]"
  [T] -> Bus Creator2/3  "Temperature [C]"
  Source2/1(Out1) -> Gain/1
  Bus Creator1/1 -> Out2/1
  [T] -> Bus Creator1/2  "Temp"
  [Q_sink] -> Bus Creator1/1  "Q_kW"
  Gain/1 -> [Q_sink]

== system DAEMOT_Lib/Electrical/Inverter_v1 ==
  In1 : Inport
  In2 : Inport  Port=2
  Bus Creator1 : BusCreator  Inputs=2
  Bus Creator2 : BusCreator  Inputs=3
  Bus Creator3 : BusCreator  Inputs=2
  Bus Selector1 : BusSelector  OutputSignals=current,voltage
  Data_Sink : $bdroot/Support Functions/Data_Sink
  Gain : Gain  Gain=1000
  Integrator1 : Integrator  InitialCondition=T_initial
  Sink : $bdroot/Support Functions/Sink
  Source1 : $bdroot/Support Functions/Source
  Source2 : $bdroot/Support Functions/Source
  Terminator : Terminator
  Thermal : MATLAB Function  TreatAsAtomicUnit=on
  Voltage_Current : MATLAB Function  TreatAsAtomicUnit=on
  Out1 : Outport  VectorParamsAs1DForOutWhenUnconnected=off
  Out2 : Outport  Port=2  VectorParamsAs1DForOutWhenUnconnected=off
  wires:
  Voltage_Current/2(I_in) -> [I_in]
  In2/1 -> Voltage_Current/3(D)
  [I_out] -> Voltage_Current/2(I_out)
  Bus Creator3/1 -> Out1/1
  In1/1 -> Bus Selector1/1  "electric"
  [I_in] -> Sink/1
  [V_out] -> Bus Creator3/2  "voltage"
  Bus Selector1/2 -> [V_in]  "<voltage>"
  Bus Selector1/1 -> Terminator/1  "<current>"
  Source1/1 -> [I_out]
  [I_out] -> Bus Creator3/1  "current"
  [V_in] -> Voltage_Current/1(V_in)
  Voltage_Current/1(V_out) -> [V_out]
  [Q_sink] -> Thermal/2(Q_sink)
  [Q] -> Thermal/1(Q)
  Integrator1/1 -> [T]
  Thermal/1(T_dot) -> Integrator1/1
  Bus Creator2/1 -> Data_Sink/1
  [V_out] -> Bus Creator2/2  "Voltage"
  [I_out] -> Bus Creator2/1  "Current"
  [T] -> Bus Creator2/3  "Temperature"
  Voltage_Current/3(Q) -> [Q]
  Source2/1 -> Gain/1
  Bus Creator1/1 -> Out2/1
  [T] -> Bus Creator1/2  "Temp"
  [Q_sink] -> Bus Creator1/1  "Q_kW"
  Gain/1 -> [Q_sink]

== system DAEMOT_Lib/Electrical/Motor ==
  In1 : Inport
  Bus Creator1 : BusCreator  Inputs=2
  Bus Creator2 : BusCreator  Inputs=3
  Bus Creator3 : BusCreator  Inputs=2
  Bus Selector1 : BusSelector  OutputSignals=current,voltage
  Current : MATLAB Function  TreatAsAtomicUnit=on
  Data_Sink : Subsystem  LoadFcn=|  InitFcn=|  mask(Data Sink){}
      LoadFcn=|
      | h      = get_param(gcb,'handle');   % Get block handle                           
      | hblock = get(h);     % Parse out handles structure
      | 
      | str = [hblock.Path(numel(bdroot)+2:end), hblock.Name];
      | str(~ismember(str,['A':'Z' 'a':'z' '0':'9' '_'])) = '';                     
      | set_param([gcb, '/global_data_goto'],'GotoTag',['gdata_',str]);
      |                                
      |                                                                                  
      | clear h hblock str
      InitFcn=|
      | h      = get_param(gcb,'handle');   % Get block handle                           
      | hblock = get(h);     % Parse out handles structure
      | 
      | str = [hblock.Path(numel(bdroot)+2:end), hblock.Name];
      | str(~ismember(str,['A':'Z' 'a':'z' '0':'9' '_'])) = '';                     
      | set_param([gcb, '/global_data_goto'],'GotoTag',['gdata_',str]);
      |                                
      |                                                                                  
      | clear h hblock str
      mask help:
      | Input to this block should be a bus signal with named signals.
      |
      | Bus signals sent to this block will be read by the Data Manager.
      | The Data Manager will handle the global routing of signals.
      |
      | This block should be placed under the mask of components.
      settings: CopyFcn=|
      | h      = get_param(gcb,'handle');   % Get block handle
      | hblock = get(h);     % Parse out handles structure
      | 
      | str = [hblock.Path(numel(bdroot)+2:end), hblock.Name];
      | str(~ismember(str,['A':'Z' 'a':'z' '0':'9' '_'])) = '';
      | set_param([gcb, '/global_data_goto'],'GotoTag',['gdata_',str]);
      | 
      | 
      | clear h hblock str
      settings: NameChangeFcn=|
      | h      = get_param(gcb,'handle');   % Get block handle
      | hblock = get(h);     % Parse out handles structure
      | 
      | str = [hblock.Path(numel(bdroot)+2:end), hblock.Name];
      | str(~ismember(str,['A':'Z' 'a':'z' '0':'9' '_'])) = '';
      | set_param([gcb, '/global_data_goto'],'GotoTag',['gdata_',str]);
      | 
      | 
      | clear h hblock str
      mask Display: text(0.25,0.5,'Data Sink')
  Gain : Gain  Gain=1000
  Integrator : Integrator  InitialCondition=I_initial
  Integrator1 : Integrator  InitialCondition=T_initial
  Integrator2 : Integrator  InitialCondition=w_initial
  Omega : MATLAB Function  TreatAsAtomicUnit=on
  Sink1 : Subsystem  LoadFcn=rev_comms_sink();  InitFcn=rev_comms_sink();  mask(Sink){}
      mask help: Used for sending data to the upstream component.
      settings: CopyFcn=rev_comms_sink();  NameChangeFcn=rev_comms_sink();
      mask Display: text(0.25,0.5,'Sink')
  Source1 : Subsystem  mask(Source){}
      mask help: Used for receiving data from the downstream component.
      mask init:
      | n_src = gcb;
      | n_src = str2num(n_src(end));
      | try
      |     rev_comms_source(n_src);
      | catch
      | 
      | end
      mask Display: text(0.25,0.5,'Source')
  Source2 : Subsystem  mask(Source){}
      mask help: Used for receiving data from the downstream component.
      mask init:
      | n_src = gcb;
      | n_src = str2num(n_src(end));
      | try
      |     rev_comms_source(n_src);
      | catch
      | 
      | end
      mask Display: text(0.25,0.5,'Source')
  Terminator : Terminator
  Thermal : MATLAB Function  TreatAsAtomicUnit=on
  Out1 : Outport
  Out2 : Outport  Port=2
  wires:
  [I] -> Bus Creator2/1  "Current [A]"
  [T_motor] -> Bus Creator3/2  "torque"
  Omega/2(T_motor) -> [T_motor]
  Integrator2/1 -> [omega]
  [T_load] -> Omega/2(T_load)
  Omega/1(omega_dot) -> Integrator2/1
  [Q_sink] -> Thermal/3(Q_sink)
  [Q_elec] -> Thermal/1(Q_elec)
  Current/2(Q_elec) -> [Q_elec]
  Integrator1/1 -> [T]
  Thermal/1(T_dot) -> Integrator1/1
  [I] -> Current/2(I_in)
  Current/1(dI_dt) -> Integrator/1
  Bus Creator3/1 -> Out1/1
  In1/1 -> Bus Selector1/1  "electric"
  [I] -> Sink1/1(In1)
  [omega] -> Bus Creator3/1  "aspeed"
  Bus Selector1/2 -> [V_in]  "<voltage>"
  Bus Selector1/1 -> Terminator/1  "<current>"
  [omega] -> Current/3(omega)
  Bus Creator2/1 -> Data_Sink/1(" ")
  [omega] -> Bus Creator2/2  "Speed [rad_s]"
  [T] -> Bus Creator2/3  "Temperature [C]"
  Integrator/1 -> Omega/1(I_in), [I]
  [V_in] -> Current/1(V_in)
  Source2/1(Out1) -> Gain/1
  Source1/1(Out1) -> [T_load]
  [omega] -> Omega/3(omega)
  Omega/3(Q_mech) -> [Q_mech]
  [Q_mech] -> Thermal/2(Q_mech)
  Bus Creator1/1 -> Out2/1
  [T] -> Bus Creator1/2  "Temp"
  [Q_sink] -> Bus Creator1/1  "Q_kW"
  Gain/1 -> [Q_sink]

== system DAEMOT_Lib/Electrical/MotorNoShaft ==
  In1 : Inport
  Bus Creator1 : BusCreator  Inputs=2
  Bus Creator2 : BusCreator  Inputs=3
  Bus Creator3 : BusCreator  Inputs=2
  Bus Selector1 : BusSelector  OutputSignals=current,voltage
  Current : MATLAB Function  TreatAsAtomicUnit=on
  Data_Sink : Subsystem  LoadFcn=|  InitFcn=|  mask(Data Sink){}
      LoadFcn=|
      | h      = get_param(gcb,'handle');   % Get block handle                           
      | hblock = get(h);     % Parse out handles structure
      | 
      | str = [hblock.Path(numel(bdroot)+2:end), hblock.Name];
      | str(~ismember(str,['A':'Z' 'a':'z' '0':'9' '_'])) = '';                     
      | set_param([gcb, '/global_data_goto'],'GotoTag',['gdata_',str]);
      |                                
      |                                                                                  
      | clear h hblock str
      InitFcn=|
      | h      = get_param(gcb,'handle');   % Get block handle                           
      | hblock = get(h);     % Parse out handles structure
      | 
      | str = [hblock.Path(numel(bdroot)+2:end), hblock.Name];
      | str(~ismember(str,['A':'Z' 'a':'z' '0':'9' '_'])) = '';                     
      | set_param([gcb, '/global_data_goto'],'GotoTag',['gdata_',str]);
      |                                
      |                                                                                  
      | clear h hblock str
      mask help:
      | Input to this block should be a bus signal with named signals.
      |
      | Bus signals sent to this block will be read by the Data Manager.
      | The Data Manager will handle the global routing of signals.
      |
      | This block should be placed under the mask of components.
      settings: CopyFcn=|
      | h      = get_param(gcb,'handle');   % Get block handle
      | hblock = get(h);     % Parse out handles structure
      | 
      | str = [hblock.Path(numel(bdroot)+2:end), hblock.Name];
      | str(~ismember(str,['A':'Z' 'a':'z' '0':'9' '_'])) = '';
      | set_param([gcb, '/global_data_goto'],'GotoTag',['gdata_',str]);
      | 
      | 
      | clear h hblock str
      settings: NameChangeFcn=|
      | h      = get_param(gcb,'handle');   % Get block handle
      | hblock = get(h);     % Parse out handles structure
      | 
      | str = [hblock.Path(numel(bdroot)+2:end), hblock.Name];
      | str(~ismember(str,['A':'Z' 'a':'z' '0':'9' '_'])) = '';
      | set_param([gcb, '/global_data_goto'],'GotoTag',['gdata_',str]);
      | 
      | 
      | clear h hblock str
      mask Display: text(0.25,0.5,'Data Sink')
  Gain : Gain  Gain=1000
  Integrator : Integrator  InitialCondition=I_initial
  Integrator1 : Integrator  InitialCondition=T_initial
  Sink1 : Subsystem  LoadFcn=rev_comms_sink();  InitFcn=rev_comms_sink();  mask(Sink){}
      mask help: Used for sending data to the upstream component.
      settings: CopyFcn=rev_comms_sink();  NameChangeFcn=rev_comms_sink();
      mask Display: text(0.25,0.5,'Sink')
  Source1 : Subsystem  mask(Source){}
      mask help: Used for receiving data from the downstream component.
      mask init:
      | n_src = gcb;
      | n_src = str2num(n_src(end));
      | try
      |     rev_comms_source(n_src);
      | catch
      | 
      | end
      mask Display: text(0.25,0.5,'Source')
  Source2 : Subsystem  mask(Source){}
      mask help: Used for receiving data from the downstream component.
      mask init:
      | n_src = gcb;
      | n_src = str2num(n_src(end));
      | try
      |     rev_comms_source(n_src);
      | catch
      | 
      | end
      mask Display: text(0.25,0.5,'Source')
  Terminator : Terminator
  Thermal : MATLAB Function  TreatAsAtomicUnit=on
  Torque : MATLAB Function  TreatAsAtomicUnit=on
  Out1 : Outport
  Out2 : Outport  Port=2
  wires:
  [I] -> Bus Creator2/1  "Current [A]"
  [tau] -> Bus Creator3/2  "torque"
  Torque/1(T_motor) -> [tau]
  [Q_sink] -> Thermal/3(Q_sink)
  [Q_elec] -> Thermal/1(Q_elec)
  Current/2(Q_elec) -> [Q_elec]
  Integrator1/1 -> [T]
  Thermal/1(T_dot) -> Integrator1/1
  [I] -> Current/2(I_in)
  Current/1(dI_dt) -> Integrator/1
  Bus Creator3/1 -> Out1/1
  In1/1 -> Bus Selector1/1  "electric"
  [I] -> Sink1/1(In1)
  [omega] -> Bus Creator3/1  "aspeed"
  Bus Selector1/2 -> [V_in]  "<voltage>"
  Bus Selector1/1 -> Terminator/1  "<current>"
  [omega] -> Current/3(omega)
  Bus Creator2/1 -> Data_Sink/1(" ")
  [tau] -> Bus Creator2/2  "Torque [Nm]"
  [T] -> Bus Creator2/3  "Temperature [C]"
  Integrator/1 -> Torque/1(I_in), [I]
  [V_in] -> Current/1(V_in)
  Source2/1(Out1) -> Gain/1
  Source1/1(Out1) -> [omega]
  [omega] -> Torque/2(omega)
  Torque/2(Q_mech) -> [Q_mech]
  [Q_mech] -> Thermal/2(Q_mech)
  Bus Creator1/1 -> Out2/1
  [T] -> Bus Creator1/2  "Temp"
  [Q_sink] -> Bus Creator1/1  "Q_kW"
  Gain/1 -> [Q_sink]

== system DAEMOT_Lib/Electrical/Resistor ==
  In1 : Inport
  In2 : Inport  Port=2
  Bus Creator1 : BusCreator  Inputs=3
  Bus Creator2 : BusCreator  Inputs=2
  Bus Creator3 : BusCreator  Inputs=2
  Bus Selector1 : BusSelector  OutputSignals=current,voltage
  Data_Sink : $bdroot/Support Functions/Data_Sink
  Electrical : MATLAB Function  TreatAsAtomicUnit=on
  Gain : Gain  Gain=1000
  Integrator1 : Integrator  InitialCondition=T_initial
  Sink1 : $bdroot/Support Functions/Sink
  Source1 : $bdroot/Support Functions/Source
  Source2 : $bdroot/Support Functions/Source
  Terminator : Terminator
  Thermal : MATLAB Function  TreatAsAtomicUnit=on
  Out1 : Outport  VectorParamsAs1DForOutWhenUnconnected=off
  Out2 : Outport  Port=2  VectorParamsAs1DForOutWhenUnconnected=off
  wires:
  In2/1 -> Electrical/3(R)
  Source2/1 -> Gain/1
  [T] -> Bus Creator1/3  "Temperature"
  Electrical/2(Q) -> [Q]
  Thermal/1(T_dot) -> Integrator1/1
  Integrator1/1 -> [T]
  [Q] -> Thermal/1(Q)
  [Q_sink] -> Thermal/2(Q_sink)
  Bus Creator1/1 -> Data_Sink/1
  [out] -> Bus Creator1/2  "Voltage"
  [in] -> Bus Creator1/1  "Current"
  [in] -> Electrical/2(in)
  [V_in] -> Electrical/1(V_in)
  Bus Creator3/1 -> Out1/1
  Electrical/1(out) -> [out]
  In1/1 -> Bus Selector1/1  "electric"
  [in] -> Sink1/1
  [out] -> Bus Creator3/2  "voltage"
  Bus Selector1/2 -> [V_in]  "<voltage>"
  Bus Selector1/1 -> Terminator/1  "<current>"
  Source1/1 -> [in]
  [in] -> Bus Creator3/1  "current"
  Bus Creator2/1 -> Out2/1
  [T] -> Bus Creator2/2  "Temp"
  [Q_sink] -> Bus Creator2/1  "Q_kW"
  Gain/1 -> [Q_sink]
